simulink model "big2"  (R2023b)
settings: Solver=VariableStepAuto  StartTime=0.0  StopTime=500  RelTol=1e-3
libraries: simulink x2, aerolibasang x2, simulink_extras x2, aerolibanim x1
(part 1 of 3)
settings Model: Creator=TADTAWAN  LastModifiedBy=TADTAWAN

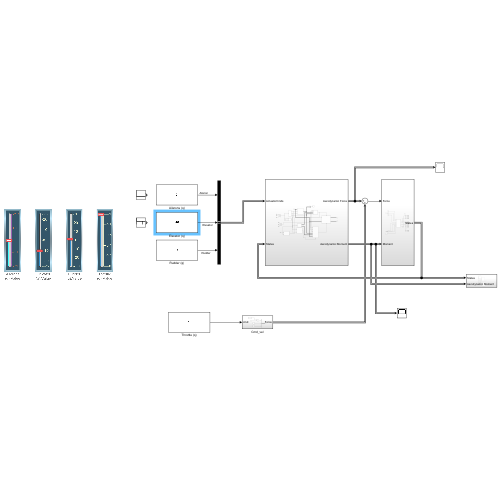
[thumbnail: Simulink's stored preview of the top-level diagram]
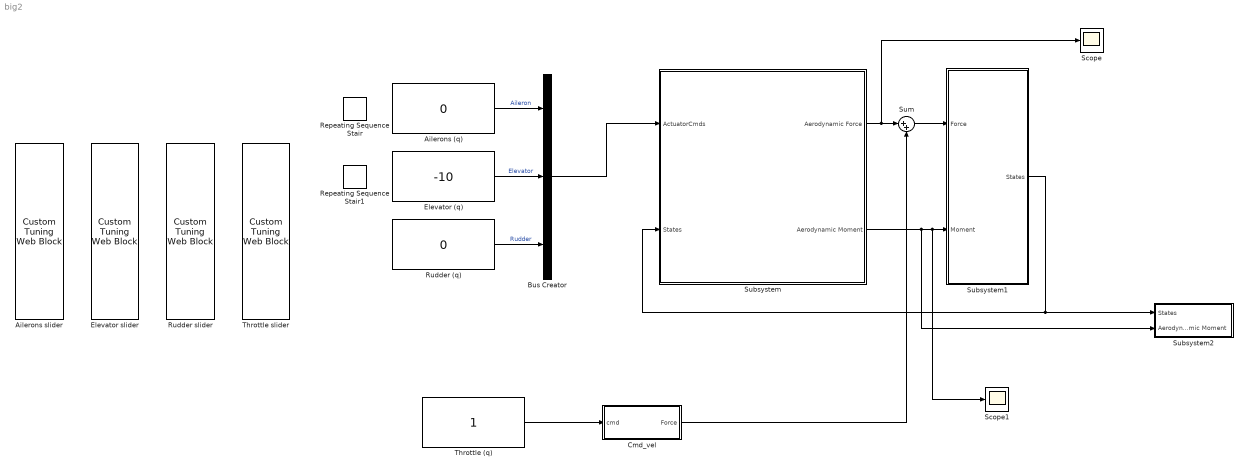
== system big2 ==
  Ailerons (q) : Constant  Value=0
  Ailerons slider : CustomTuningWebBlock  LabelPosition=Bottom  ShowInitialText=on  Configuration="{\"components\":[{\"name\":\"LinearScaleComponent\",\"settings\":{\"bounds\":{\"max\":21.5,\"min\":-21.5,\"tickInterval\":\"auto\"},\"internalTickHeightScaleFactor\":0.5,\"labelColor\":[181,82,43],\"labelFont\":{\"font\":\"Arial\",\"fontSize\":12},\"labelOffset\":0.05,\"labelTransparency\":1,\"needleImage\":{\"size\":[596,842],\"src\":\"data:image\\/svg+xml;base64,PD94bWwgdmVyc2lvbj0iMS4wIiBlbmNvZGluZz0idXRmLTgiPz4NCjwhLS0gR2VuZXJhdG9yOiBBZG9iZSBJbGx1c3RyYXRvciAyNS4wLjAsIFNWRyBFeHBvcnQgUGx1Zy1JbiAuIFNWRyBWZXJzaW9uOiA2LjAwIEJ1aWxkIDApICAtLT4NCjxzdmcgdmVyc2lvbj0iMS4xIg0KCSBpZD0ic3ZnOCIgeG1sbnM6Y2M9Imh0dHA6Ly9jcmVhdGl2ZWNvbW1vbnMub3JnL25zIyIgeG1sbnM6ZGM9Imh0dHA6Ly9wdXJsLm9yZy9kYy9lbGVtZW50cy8xLjEvIiB4bWxuczppbmtzY2FwZT0iaHR0cDovL3d3dy5pbmtzY2FwZS5vcmcvbmFtZXNw ...(+2420 chars)\",\"srcOrientation\":\"horizontal\"},\"needleOffset\":[0.0642123287671233,-0.8044596912521441],\"needleSize\":{\"height\":0.07668067226890757,\"width\":0.4337797619047619},\"position\":[0.03623949579831933,0.2829861111111111,0.6088789682539683,0.9196428571428571],\"referencePoint\":\"auto\",\"scaleColors\":[],\"scaleColorsSize\":0.2,\"scaleDirection\":\"BT\",\"showLabels\":1,\"showMinorTicks\":0,\"showSpanLine\":1,\"showTicks\":1,\"tickColor\":[150,61,168],\"tickTransparency\":1,\"valueBarColor\":[15,255,255],\"valueBarOffset\":-0.27,\"valueBarSize\":0.1,\"valueBarTransparency\":1}},{\"name\":\"BackgroundImageComponent\",\"settings\":{\"image\":{\"size\":[380,101],\"src\":\"data:image\\/svg+xml;base64,PHN2ZyB4bWxucz0iaHR0cDovL3d3dy53My5vcmcvMjAwMC9zdmciIHhtbG5zOnhsaW5rPSJodHRwOi8vd3d3LnczLm9yZy8xOTk5L3hsaW5rIiB2aWV3Qm94PSIwIDAgMzgwIDEwMSI+PGRlZnM+PHN0eWxlPi5jbHMtMXtmaWxsOiMwMDJiNDI7fS5jbHMtMntmaWxsOiM0MjcwODI7fS5jbHMtM3tmaWxsOnVybCgjcmFkaWFsLWdyYWRpZW50KTt9LmNscy00e2ZpbGw6I2M4YzhjODtzdHJva2U6IzAwMDt9PC9zdHlsZT48cmFkaWFsR3JhZGllbnQgaWQ9InJhZGlhbC1ncmFkaWVudCIgY3g9IjE5MCIgY3k9IjUwLjUiIHI9IjI2OS4yMSIgZ3JhZGllbnRVbml0cz0idXNlclNwYWNlT25Vc2UiPjxzdG9wIG9mZnNldD0iMC4wMSIgc3RvcC1jb2xvcj0iIzNlNGY1OCIvPjxzdG9wIG9mZnNldD0iMC4wNiIgc3RvcC1jb2xvcj0iIzQ0NTc2MSIvPjxzdG9wIG9mZnNldD0iMC4xNSIgc3RvcC1jb2xvcj0iIzU1NmE3NiIvPjxzdG9wIG9mZnNldD0iMC4yNSIgc3RvcC1jb2xvcj0iIzZkODg5NSIvPjxzdG9wIG9mZnNldD0iMC4zOCIgc3RvcC1jb2xvcj0iIzhmYjJjMyIvPjxzdG9wIG9mZnNldD0iMC41MiIgc3RvcC1jb2xvcj0iI2I2ZTRmYSIvPjxzdG9wIG9mZnNldD0iMSIgc3RvcC1jb2xvcj0iIzE1NDY1NyIvPjwvcmFkaWFsR3JhZGllbnQ+PC9kZWZzPjxnIGlkPSJmcmFtZSI+PGcgaWQ9IkxheWVyXzIiIGRhdGEtbmFtZT0iTGF5ZXIgMiI+PGcgaWQ9IkxheWVyXzEtMiIgZGF0YS1uYW1lPSJMYXllciAxLTIiPjxyZWN0IGlkPSJyZWN0MTAzNiIgY2xhc3M9ImNscy0xIiB4PSIxMSIgeT0iMTEiIHdpZHRoPSIzNTgiIGhlaWdodD0iNzkiLz48cGF0aCBpZD0icGF0aDEwMzgiIGNsYXNzPSJjbHMtMiIgZD0iTTgsOFY5M0gzNzJWOFpNMzY5LDkwSDExVjExSDM2OVoiLz48cGF0aCBpZD0icGF0aDEwNDAiIGNsYXNzPSJjbHMtMyIgZD0iTTAsMFYxMDFIMzgwVjBaTTM3Miw5M0g4VjhIMzcyWiIvPjwvZz48L2c+PC9nPjxnIGlkPSJ0cmFjayI+PHBhdGggaWQ9InJlY3QxNjExIiBjbGFzcz0iY2xzLTQiIGQ9Ik0zMy4zNywyNi41OUgzNDYuNjNjNCwwLDcuMjUsMi42LDcuMjUsNS44MWgwYzAsMy4yMS0zLjI1LDUuODItNy4yNSw1LjgySDMzLjM3Yy00LDAtNy4yNS0yLjYxLTcuMjUtNS44MmgwQzI2LjEyLDI5LjE5LDI5LjM3LDI2LjU5LDMzLjM3LDI2LjU5WiIvPjwvZz48L3N2Zz4=\",\"srcOrientation\":\"horizontal\"},\"position\":[0,0,1,1],\"scaleMode\":\"0\"}},{\"name\":\"ForegroundImageComponent\",\"settings\":{\"image\":{\"size\":[0,0],\"src\":\"default\",\"srcOrientation\":[]},\"isForeground\":1,\"position\":[0,0,1,1],\"scaleMode\":\"0\"}}],\"settings\":{\"BindingType\":\"param\",\"aspectRatio\":3.7777777777777777,\"backgroundColor\":[0,0,0,\"1\"],\"backgroundOffset\":0,\"backgroundOpacity\":1,\"fixedAspectRatio\":\"on\",\"foregroundColor\":[252,252,196],\"orientation\":\"vertical\",\"showBackgroundColor\":false,\"value\":0,\"version\":\"R2023a\"},\"type\":\"LinearGauge\"}"
  Bus Creator : BusCreator  Inputs=3
  Cmd_vel : Subsystem
  Elevator (q) : Constant  Value=-10
  Elevator slider : CustomTuningWebBlock  LabelPosition=Bottom  ShowInitialText=on  Configuration="{\"components\":[{\"name\":\"LinearScaleComponent\",\"settings\":{\"bounds\":{\"max\":25,\"min\":-25,\"tickInterval\":\"auto\"},\"internalTickHeightScaleFactor\":0.5,\"labelColor\":[255,255,200],\"labelFont\":{\"font\":\"Arial\",\"fontSize\":12},\"labelOffset\":0.05,\"labelTransparency\":1,\"needleImage\":{\"size\":[596,842],\"src\":\"data:image\\/svg+xml;base64,PD94bWwgdmVyc2lvbj0iMS4wIiBlbmNvZGluZz0idXRmLTgiPz4NCjwhLS0gR2VuZXJhdG9yOiBBZG9iZSBJbGx1c3RyYXRvciAyNS4wLjAsIFNWRyBFeHBvcnQgUGx1Zy1JbiAuIFNWRyBWZXJzaW9uOiA2LjAwIEJ1aWxkIDApICAtLT4NCjxzdmcgdmVyc2lvbj0iMS4xIg0KCSBpZD0ic3ZnOCIgeG1sbnM6Y2M9Imh0dHA6Ly9jcmVhdGl2ZWNvbW1vbnMub3JnL25zIyIgeG1sbnM6ZGM9Imh0dHA6Ly9wdXJsLm9yZy9kYy9lbGVtZW50cy8xLjEvIiB4bWxuczppbmtzY2FwZT0iaHR0cDovL3d3dy5pbmtzY2FwZS5vcmcvbmFtZXNw ...(+2420 chars)\",\"srcOrientation\":\"horizontal\"},\"needleOffset\":[0.0642123287671233,-0.8044596912521441],\"needleSize\":{\"height\":0.07668067226890757,\"width\":0.4337797619047619},\"position\":[0.03623949579831933,0.2829861111111111,0.6088789682539683,0.9196428571428571],\"referencePoint\":\"auto\",\"scaleColors\":[],\"scaleColorsSize\":0.2,\"scaleDirection\":\"BT\",\"showLabels\":1,\"showMinorTicks\":0,\"showSpanLine\":1,\"showTicks\":1,\"tickColor\":[252,252,197],\"tickTransparency\":1,\"valueBarColor\":[0,114,189],\"valueBarOffset\":-0.27,\"valueBarSize\":0.1,\"valueBarTransparency\":1}},{\"name\":\"BackgroundImageComponent\",\"settings\":{\"image\":{\"size\":[380,101],\"src\":\"data:image\\/svg+xml;base64,PHN2ZyB4bWxucz0iaHR0cDovL3d3dy53My5vcmcvMjAwMC9zdmciIHhtbG5zOnhsaW5rPSJodHRwOi8vd3d3LnczLm9yZy8xOTk5L3hsaW5rIiB2aWV3Qm94PSIwIDAgMzgwIDEwMSI+PGRlZnM+PHN0eWxlPi5jbHMtMXtmaWxsOiMwMDJiNDI7fS5jbHMtMntmaWxsOiM0MjcwODI7fS5jbHMtM3tmaWxsOnVybCgjcmFkaWFsLWdyYWRpZW50KTt9LmNscy00e2ZpbGw6I2M4YzhjODtzdHJva2U6IzAwMDt9PC9zdHlsZT48cmFkaWFsR3JhZGllbnQgaWQ9InJhZGlhbC1ncmFkaWVudCIgY3g9IjE5MCIgY3k9IjUwLjUiIHI9IjI2OS4yMSIgZ3JhZGllbnRVbml0cz0idXNlclNwYWNlT25Vc2UiPjxzdG9wIG9mZnNldD0iMC4wMSIgc3RvcC1jb2xvcj0iIzNlNGY1OCIvPjxzdG9wIG9mZnNldD0iMC4wNiIgc3RvcC1jb2xvcj0iIzQ0NTc2MSIvPjxzdG9wIG9mZnNldD0iMC4xNSIgc3RvcC1jb2xvcj0iIzU1NmE3NiIvPjxzdG9wIG9mZnNldD0iMC4yNSIgc3RvcC1jb2xvcj0iIzZkODg5NSIvPjxzdG9wIG9mZnNldD0iMC4zOCIgc3RvcC1jb2xvcj0iIzhmYjJjMyIvPjxzdG9wIG9mZnNldD0iMC41MiIgc3RvcC1jb2xvcj0iI2I2ZTRmYSIvPjxzdG9wIG9mZnNldD0iMSIgc3RvcC1jb2xvcj0iIzE1NDY1NyIvPjwvcmFkaWFsR3JhZGllbnQ+PC9kZWZzPjxnIGlkPSJmcmFtZSI+PGcgaWQ9IkxheWVyXzIiIGRhdGEtbmFtZT0iTGF5ZXIgMiI+PGcgaWQ9IkxheWVyXzEtMiIgZGF0YS1uYW1lPSJMYXllciAxLTIiPjxyZWN0IGlkPSJyZWN0MTAzNiIgY2xhc3M9ImNscy0xIiB4PSIxMSIgeT0iMTEiIHdpZHRoPSIzNTgiIGhlaWdodD0iNzkiLz48cGF0aCBpZD0icGF0aDEwMzgiIGNsYXNzPSJjbHMtMiIgZD0iTTgsOFY5M0gzNzJWOFpNMzY5LDkwSDExVjExSDM2OVoiLz48cGF0aCBpZD0icGF0aDEwNDAiIGNsYXNzPSJjbHMtMyIgZD0iTTAsMFYxMDFIMzgwVjBaTTM3Miw5M0g4VjhIMzcyWiIvPjwvZz48L2c+PC9nPjxnIGlkPSJ0cmFjayI+PHBhdGggaWQ9InJlY3QxNjExIiBjbGFzcz0iY2xzLTQiIGQ9Ik0zMy4zNywyNi41OUgzNDYuNjNjNCwwLDcuMjUsMi42LDcuMjUsNS44MWgwYzAsMy4yMS0zLjI1LDUuODItNy4yNSw1LjgySDMzLjM3Yy00LDAtNy4yNS0yLjYxLTcuMjUtNS44MmgwQzI2LjEyLDI5LjE5LDI5LjM3LDI2LjU5LDMzLjM3LDI2LjU5WiIvPjwvZz48L3N2Zz4=\",\"srcOrientation\":\"horizontal\"},\"position\":[0,0,1,1],\"scaleMode\":\"0\"}},{\"name\":\"ForegroundImageComponent\",\"settings\":{\"image\":{\"size\":[0,0],\"src\":\"default\",\"srcOrientation\":[]},\"isForeground\":1,\"position\":[0,0,1,1],\"scaleMode\":\"0\"}}],\"settings\":{\"BindingType\":\"param\",\"aspectRatio\":3.7777777777777777,\"backgroundColor\":[0,0,0,\"1\"],\"backgroundOffset\":0,\"backgroundOpacity\":1,\"fixedAspectRatio\":\"on\",\"foregroundColor\":[252,252,196],\"orientation\":\"vertical\",\"showBackgroundColor\":false,\"value\":0,\"version\":\"R2023a\"},\"type\":\"LinearGauge\"}"
  Repeating Sequence Stair : simulink/Sources/Repeating Sequence Stair  OutValues=[0 0 0 0 0 0 0 0 0 0 0 0 0 0 0 0 0 0 0 0 0 0 0 0 0 0 0 0 0 0 0 0 0].'  tsamp=8  OutMin=[]  OutMax=[]  OutDataTypeStr=double  OutputDataTypeScalingMode=double  OutDataType=fixdt(0,8)  ConRadixGroup=Best Precision: Vector-wise  OutScaling=2^-12
  Repeating Sequence Stair1 : simulink/Sources/Repeating Sequence Stair  OutValues=[25 0 0 0 0 0 0 0 0 0 0 0 0 0 0 0 0 0 0 0 0 0 0 0 0 0 0 0 0 -25 0 0 0 0 0 0 0 0 0 0 0 0 0 0 0].'  tsamp=5  OutMin=[]  OutMax=[]  OutDataTypeStr=double  OutputDataTypeScalingMode=double  OutDataType=fixdt(0,8)  ConRadixGroup=Best Precision: Vector-wise  OutScaling=2^-12
  Rudder (q) : Constant  Value=0
  Rudder slider : CustomTuningWebBlock  LabelPosition=Bottom  ShowInitialText=on  Configuration="{\"components\":[{\"name\":\"LinearScaleComponent\",\"settings\":{\"bounds\":{\"max\":30,\"min\":-30,\"tickInterval\":\"auto\"},\"internalTickHeightScaleFactor\":0.5,\"labelColor\":[255,255,200],\"labelFont\":{\"font\":\"Arial\",\"fontSize\":12},\"labelOffset\":0.05,\"labelTransparency\":1,\"needleImage\":{\"size\":[596,842],\"src\":\"data:image\\/svg+xml;base64,PD94bWwgdmVyc2lvbj0iMS4wIiBlbmNvZGluZz0idXRmLTgiPz4NCjwhLS0gR2VuZXJhdG9yOiBBZG9iZSBJbGx1c3RyYXRvciAyNS4wLjAsIFNWRyBFeHBvcnQgUGx1Zy1JbiAuIFNWRyBWZXJzaW9uOiA2LjAwIEJ1aWxkIDApICAtLT4NCjxzdmcgdmVyc2lvbj0iMS4xIg0KCSBpZD0ic3ZnOCIgeG1sbnM6Y2M9Imh0dHA6Ly9jcmVhdGl2ZWNvbW1vbnMub3JnL25zIyIgeG1sbnM6ZGM9Imh0dHA6Ly9wdXJsLm9yZy9kYy9lbGVtZW50cy8xLjEvIiB4bWxuczppbmtzY2FwZT0iaHR0cDovL3d3dy5pbmtzY2FwZS5vcmcvbmFtZXNw ...(+2420 chars)\",\"srcOrientation\":\"Right\"},\"needleOffset\":[-0.21513706793802145,-0.7877922077922078],\"needleSize\":{\"height\":0.07666301169590643,\"width\":0.43370508054522927},\"position\":[0.03623949579831933,0.2829861111111111,0.6088789682539683,0.9196428571428571],\"referencePoint\":\"auto\",\"scaleColors\":[],\"scaleColorsSize\":0.2,\"scaleDirection\":\"BT\",\"showLabels\":1,\"showMinorTicks\":0,\"showSpanLine\":1,\"showTicks\":1,\"tickColor\":[252,252,197],\"tickTransparency\":1,\"valueBarColor\":[0,114,189],\"valueBarOffset\":-0.27,\"valueBarSize\":0.1,\"valueBarTransparency\":1}},{\"name\":\"BackgroundImageComponent\",\"settings\":{\"image\":{\"size\":[380,101],\"src\":\"data:image\\/svg+xml;base64,PHN2ZyB4bWxucz0iaHR0cDovL3d3dy53My5vcmcvMjAwMC9zdmciIHhtbG5zOnhsaW5rPSJodHRwOi8vd3d3LnczLm9yZy8xOTk5L3hsaW5rIiB2aWV3Qm94PSIwIDAgMzgwIDEwMSI+PGRlZnM+PHN0eWxlPi5jbHMtMXtmaWxsOiMwMDJiNDI7fS5jbHMtMntmaWxsOiM0MjcwODI7fS5jbHMtM3tmaWxsOnVybCgjcmFkaWFsLWdyYWRpZW50KTt9LmNscy00e2ZpbGw6I2M4YzhjODtzdHJva2U6IzAwMDt9PC9zdHlsZT48cmFkaWFsR3JhZGllbnQgaWQ9InJhZGlhbC1ncmFkaWVudCIgY3g9IjE5MCIgY3k9IjUwLjUiIHI9IjI2OS4yMSIgZ3JhZGllbnRVbml0cz0idXNlclNwYWNlT25Vc2UiPjxzdG9wIG9mZnNldD0iMC4wMSIgc3RvcC1jb2xvcj0iIzNlNGY1OCIvPjxzdG9wIG9mZnNldD0iMC4wNiIgc3RvcC1jb2xvcj0iIzQ0NTc2MSIvPjxzdG9wIG9mZnNldD0iMC4xNSIgc3RvcC1jb2xvcj0iIzU1NmE3NiIvPjxzdG9wIG9mZnNldD0iMC4yNSIgc3RvcC1jb2xvcj0iIzZkODg5NSIvPjxzdG9wIG9mZnNldD0iMC4zOCIgc3RvcC1jb2xvcj0iIzhmYjJjMyIvPjxzdG9wIG9mZnNldD0iMC41MiIgc3RvcC1jb2xvcj0iI2I2ZTRmYSIvPjxzdG9wIG9mZnNldD0iMSIgc3RvcC1jb2xvcj0iIzE1NDY1NyIvPjwvcmFkaWFsR3JhZGllbnQ+PC9kZWZzPjxnIGlkPSJmcmFtZSI+PGcgaWQ9IkxheWVyXzIiIGRhdGEtbmFtZT0iTGF5ZXIgMiI+PGcgaWQ9IkxheWVyXzEtMiIgZGF0YS1uYW1lPSJMYXllciAxLTIiPjxyZWN0IGlkPSJyZWN0MTAzNiIgY2xhc3M9ImNscy0xIiB4PSIxMSIgeT0iMTEiIHdpZHRoPSIzNTgiIGhlaWdodD0iNzkiLz48cGF0aCBpZD0icGF0aDEwMzgiIGNsYXNzPSJjbHMtMiIgZD0iTTgsOFY5M0gzNzJWOFpNMzY5LDkwSDExVjExSDM2OVoiLz48cGF0aCBpZD0icGF0aDEwNDAiIGNsYXNzPSJjbHMtMyIgZD0iTTAsMFYxMDFIMzgwVjBaTTM3Miw5M0g4VjhIMzcyWiIvPjwvZz48L2c+PC9nPjxnIGlkPSJ0cmFjayI+PHBhdGggaWQ9InJlY3QxNjExIiBjbGFzcz0iY2xzLTQiIGQ9Ik0zMy4zNywyNi41OUgzNDYuNjNjNCwwLDcuMjUsMi42LDcuMjUsNS44MWgwYzAsMy4yMS0zLjI1LDUuODItNy4yNSw1LjgySDMzLjM3Yy00LDAtNy4yNS0yLjYxLTcuMjUtNS44MmgwQzI2LjEyLDI5LjE5LDI5LjM3LDI2LjU5LDMzLjM3LDI2LjU5WiIvPjwvZz48L3N2Zz4=\",\"srcOrientation\":\"horizontal\"},\"position\":[0,0,1,1],\"scaleMode\":\"0\"}},{\"name\":\"ForegroundImageComponent\",\"settings\":{\"image\":{\"size\":[0,0],\"src\":\"default\",\"srcOrientation\":[]},\"isForeground\":1,\"position\":[0,0,1,1],\"scaleMode\":\"0\"}}],\"settings\":{\"BindingType\":\"param\",\"aspectRatio\":3.7777777777777777,\"backgroundColor\":[0,0,0,\"1\"],\"backgroundOffset\":0,\"backgroundOpacity\":1,\"fixedAspectRatio\":\"on\",\"foregroundColor\":[252,252,196],\"orientation\":\"vertical\",\"showBackgroundColor\":false,\"value\":0,\"version\":\"R2023a\"},\"type\":\"LinearGauge\"}"
  Scope : Scope
  Scope1 : Scope
  Subsystem : Subsystem
  Subsystem1 : Subsystem
  Subsystem2 : Subsystem
  Sum : Sum  Inputs=|++
  Throttle (q) : Constant
  Throttle slider : CustomTuningWebBlock  LabelPosition=Bottom  ShowInitialText=on  Configuration="{\"components\":[{\"name\":\"LinearScaleComponent\",\"settings\":{\"bounds\":{\"max\":1,\"min\":0,\"tickInterval\":\"auto\"},\"internalTickHeightScaleFactor\":0.5,\"labelColor\":[255,255,200],\"labelFont\":{\"font\":\"Arial\",\"fontSize\":12},\"labelOffset\":0.05,\"labelTransparency\":1,\"needleImage\":{\"size\":[596,842],\"src\":\"data:image\\/svg+xml;base64,PD94bWwgdmVyc2lvbj0iMS4wIiBlbmNvZGluZz0idXRmLTgiPz4NCjwhLS0gR2VuZXJhdG9yOiBBZG9iZSBJbGx1c3RyYXRvciAyNS4wLjAsIFNWRyBFeHBvcnQgUGx1Zy1JbiAuIFNWRyBWZXJzaW9uOiA2LjAwIEJ1aWxkIDApICAtLT4NCjxzdmcgdmVyc2lvbj0iMS4xIg0KCSBpZD0ic3ZnOCIgeG1sbnM6Y2M9Imh0dHA6Ly9jcmVhdGl2ZWNvbW1vbnMub3JnL25zIyIgeG1sbnM6ZGM9Imh0dHA6Ly9wdXJsLm9yZy9kYy9lbGVtZW50cy8xLjEvIiB4bWxuczppbmtzY2FwZT0iaHR0cDovL3d3dy5pbmtzY2FwZS5vcmcvbmFtZXNw ...(+2420 chars)\",\"srcOrientation\":\"horizontal\"},\"needleOffset\":[0.0642123287671233,-0.8044596912521441],\"needleSize\":{\"height\":0.07668067226890757,\"width\":0.4337797619047619},\"position\":[0.03623949579831933,0.2829861111111111,0.6088789682539683,0.9196428571428571],\"referencePoint\":\"auto\",\"scaleColors\":[],\"scaleColorsSize\":0.2,\"scaleDirection\":\"BT\",\"showLabels\":1,\"showMinorTicks\":0,\"showSpanLine\":1,\"showTicks\":1,\"tickColor\":[252,252,197],\"tickTransparency\":1,\"valueBarColor\":[0,114,189],\"valueBarOffset\":-0.27,\"valueBarSize\":0.1,\"valueBarTransparency\":1}},{\"name\":\"BackgroundImageComponent\",\"settings\":{\"image\":{\"size\":[380,101],\"src\":\"data:image\\/svg+xml;base64,PHN2ZyB4bWxucz0iaHR0cDovL3d3dy53My5vcmcvMjAwMC9zdmciIHhtbG5zOnhsaW5rPSJodHRwOi8vd3d3LnczLm9yZy8xOTk5L3hsaW5rIiB2aWV3Qm94PSIwIDAgMzgwIDEwMSI+PGRlZnM+PHN0eWxlPi5jbHMtMXtmaWxsOiMwMDJiNDI7fS5jbHMtMntmaWxsOiM0MjcwODI7fS5jbHMtM3tmaWxsOnVybCgjcmFkaWFsLWdyYWRpZW50KTt9LmNscy00e2ZpbGw6I2M4YzhjODtzdHJva2U6IzAwMDt9PC9zdHlsZT48cmFkaWFsR3JhZGllbnQgaWQ9InJhZGlhbC1ncmFkaWVudCIgY3g9IjE5MCIgY3k9IjUwLjUiIHI9IjI2OS4yMSIgZ3JhZGllbnRVbml0cz0idXNlclNwYWNlT25Vc2UiPjxzdG9wIG9mZnNldD0iMC4wMSIgc3RvcC1jb2xvcj0iIzNlNGY1OCIvPjxzdG9wIG9mZnNldD0iMC4wNiIgc3RvcC1jb2xvcj0iIzQ0NTc2MSIvPjxzdG9wIG9mZnNldD0iMC4xNSIgc3RvcC1jb2xvcj0iIzU1NmE3NiIvPjxzdG9wIG9mZnNldD0iMC4yNSIgc3RvcC1jb2xvcj0iIzZkODg5NSIvPjxzdG9wIG9mZnNldD0iMC4zOCIgc3RvcC1jb2xvcj0iIzhmYjJjMyIvPjxzdG9wIG9mZnNldD0iMC41MiIgc3RvcC1jb2xvcj0iI2I2ZTRmYSIvPjxzdG9wIG9mZnNldD0iMSIgc3RvcC1jb2xvcj0iIzE1NDY1NyIvPjwvcmFkaWFsR3JhZGllbnQ+PC9kZWZzPjxnIGlkPSJmcmFtZSI+PGcgaWQ9IkxheWVyXzIiIGRhdGEtbmFtZT0iTGF5ZXIgMiI+PGcgaWQ9IkxheWVyXzEtMiIgZGF0YS1uYW1lPSJMYXllciAxLTIiPjxyZWN0IGlkPSJyZWN0MTAzNiIgY2xhc3M9ImNscy0xIiB4PSIxMSIgeT0iMTEiIHdpZHRoPSIzNTgiIGhlaWdodD0iNzkiLz48cGF0aCBpZD0icGF0aDEwMzgiIGNsYXNzPSJjbHMtMiIgZD0iTTgsOFY5M0gzNzJWOFpNMzY5LDkwSDExVjExSDM2OVoiLz48cGF0aCBpZD0icGF0aDEwNDAiIGNsYXNzPSJjbHMtMyIgZD0iTTAsMFYxMDFIMzgwVjBaTTM3Miw5M0g4VjhIMzcyWiIvPjwvZz48L2c+PC9nPjxnIGlkPSJ0cmFjayI+PHBhdGggaWQ9InJlY3QxNjExIiBjbGFzcz0iY2xzLTQiIGQ9Ik0zMy4zNywyNi41OUgzNDYuNjNjNCwwLDcuMjUsMi42LDcuMjUsNS44MWgwYzAsMy4yMS0zLjI1LDUuODItNy4yNSw1LjgySDMzLjM3Yy00LDAtNy4yNS0yLjYxLTcuMjUtNS44MmgwQzI2LjEyLDI5LjE5LDI5LjM3LDI2LjU5LDMzLjM3LDI2LjU5WiIvPjwvZz48L3N2Zz4=\",\"srcOrientation\":\"horizontal\"},\"position\":[0,0,1,1],\"scaleMode\":\"0\"}},{\"name\":\"ForegroundImageComponent\",\"settings\":{\"image\":{\"size\":[0,0],\"src\":\"default\",\"srcOrientation\":[]},\"isForeground\":1,\"position\":[0,0,1,1],\"scaleMode\":\"0\"}}],\"settings\":{\"BindingType\":\"param\",\"aspectRatio\":3.7777777777777777,\"backgroundColor\":[0,0,0,\"1\"],\"backgroundOffset\":0,\"backgroundOpacity\":1,\"fixedAspectRatio\":\"on\",\"foregroundColor\":[252,252,196],\"orientation\":\"vertical\",\"showBackgroundColor\":false,\"value\":0,\"version\":\"R2023a\"},\"type\":\"LinearGauge\"}"
  wires:
  Throttle (q)/1 -> Cmd_vel/1(cmd)
  Bus Creator/1 -> Subsystem/1(ActuatorCmds)
  Subsystem1/1(States) -> Subsystem/2(States), Subsystem2/1(States)
  Cmd_vel/1(Force) -> Sum/2
  Sum/1 -> Subsystem1/1(Force)
  Rudder (q)/1 -> Bus Creator/3  "Rudder"
  Subsystem/1(Aerodynamic Force) -> Scope/1, Sum/1
  Subsystem/2(Aerodynamic Moment) -> Subsystem2/2(Aerodynamic Moment), Scope1/1, Subsystem1/2(Moment)
  Elevator (q)/1 -> Bus Creator/2  "Elevator"
  Ailerons (q)/1 -> Bus Creator/1  "Aileron"

== system big2/Cmd_vel ==
  cmd : Inport
  Bus Creator : BusCreator  Inputs=3
  Constant : Constant  Value=0
  Constant1 : Constant  Value=0
  Engine Power : Constant  Value=20500
  F_x : Product
  Force : Outport
  wires:
  Engine Power/1 -> F_x/1
  cmd/1 -> F_x/2
  F_x/1 -> Bus Creator/1  "F_x"
  Constant/1 -> Bus Creator/2  "F_y"
  Constant1/1 -> Bus Creator/3  "F_z"
  Bus Creator/1 -> Force/1

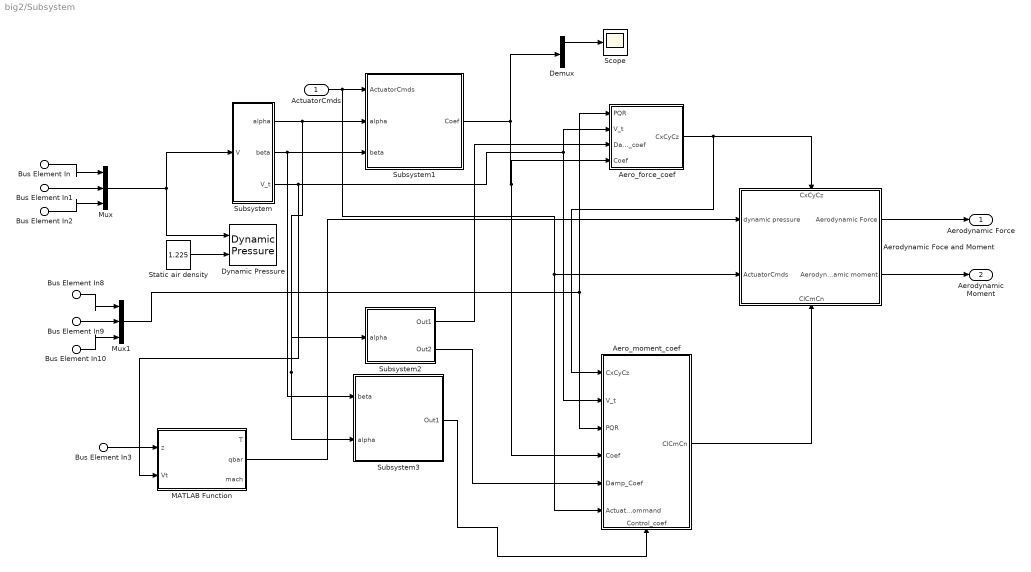
== system big2/Subsystem ==
  ActuatorCmds : Inport
  Bus Element In : Inport  Port=2  PortName=States  Element=U
  Bus Element In1 : Inport  Port=2  PortName=States  Element=V
  Bus Element In2 : Inport  Port=2  PortName=States  Element=W
  Bus Element In8 : Inport  Port=2  PortName=States  Element=p
  Bus Element In9 : Inport  Port=2  PortName=States  Element=q
  Bus Element In10 : Inport  Port=2  PortName=States  Element=r
  Bus Element In3 : Inport  Port=2  PortName=States  Element=Ze
  Aero_force_coef : Subsystem
  Aero_moment_coef : Subsystem
      settings: PortSchema="{\"entries\":[{\"content\":{\"sides\":[{\"content\":{\"connectorIds\":[\"In1\",\"In2\",\"In3\",\"In4\",\"In5\",\"In6\"]},\"type\":\"ConnectorPlacement.EquallySpacedRectSide\",\"uuid\":\"17debfaa-879f-41a8-9d58-1f255e45b172\"},{\"content\":{\"connectorIds\":[\"Out1\"],\"side\":\"RIGHT\"},\"type\":\"ConnectorPlacement.EquallySpacedRectSide\",\"uuid\":\"f07a405c-0f85-43ee-be51-ba40d2608d18\"},{\"content\":{\"side\":\"TOP\"},\"type\":\"ConnectorPlacement.EquallySpacedRectSide\",\"uuid\":\"8673e22a-5761-41aa-9cd5-8d56fc2beb8a\"},{\"content\":{\"connectorIds\":[\"In7\"],\"side\":\"BOTTOM\"},\"type\":\"ConnectorPlacement.EquallySpacedRectSide\",\"uuid\":\"a74aac7f-3bc3-4068-9fca-4bb700d9041f\"}]},\"type\":\"ConnectorPlacement.EquallySpacedConnector\",\"uuid\":\"42287ef6-e7dd-4b60-8942-44cb4f2566c7\"}],\"packageUris\":[\"http://schema.mathworks.com/mf0/Connector/R2020b\"],\"version\":\"1.0\"}"
  Aerodynamic Foce and Moment : Subsystem
      settings: PortSchema="{\"entries\":[{\"content\":{\"sides\":[{\"content\":{\"connectorIds\":[\"In1\",\"In2\"]},\"type\":\"ConnectorPlacement.EquallySpacedRectSide\",\"uuid\":\"ab71a591-92c3-4a8b-addc-090922ce6fb0\"},{\"content\":{\"connectorIds\":[\"Out1\",\"Out2\"],\"side\":\"RIGHT\"},\"type\":\"ConnectorPlacement.EquallySpacedRectSide\",\"uuid\":\"1820ed69-80c2-44ce-a026-73df58491777\"},{\"content\":{\"connectorIds\":[\"In3\"],\"side\":\"TOP\"},\"type\":\"ConnectorPlacement.EquallySpacedRectSide\",\"uuid\":\"870b67ff-c9d8-4b48-8001-55133f95ea6a\"},{\"content\":{\"connectorIds\":[\"In4\"],\"side\":\"BOTTOM\"},\"type\":\"ConnectorPlacement.EquallySpacedRectSide\",\"uuid\":\"51f11529-3a1c-4e22-ab27-30b6bff5f544\"}]},\"type\":\"ConnectorPlacement.EquallySpacedConnector\",\"uuid\":\"5a950543-611d-42e3-87a9-2998e260972e\"}],\"packageUris\":[\"http://schema.mathworks.com/mf0/Connector/R2020b\"],\"version\":\"1.0\"}"
  Demux : Demux  Outputs=6
  Dynamic Pressure : aerolibasang/Dynamic Pressure
  MATLAB Function : MATLAB Function  TreatAsAtomicUnit=on
  Mux : Mux  Inputs=3
  Mux1 : Mux  Inputs=3
  Scope : Scope
  Static air density : Constant  Value=1.225
  Subsystem : Subsystem
  Subsystem1 : Subsystem
  Subsystem2 : Subsystem
  Subsystem3 : Subsystem
  Aerodynamic Force : Outport
  Aerodynamic Moment : Outport  Port=2
  wires:
  Bus Element In1/1 -> Mux/2
  Bus Element In/1 -> Mux/1
  Bus Element In2/1 -> Mux/3
  Mux/1 -> Dynamic Pressure/1, Subsystem/1(V)
  ActuatorCmds/1 -> Aerodynamic Foce and Moment/2(ActuatorCmds), Aero_moment_coef/6(Actuatorcommand), Subsystem1/1(ActuatorCmds)
  Static air density/1 -> Dynamic Pressure/2
  Subsystem1/1(Coef) -> Aero_moment_coef/4(Coef), Aero_force_coef/4(Coef), Demux/1
  Aerodynamic Foce and Moment/1(Aerodynamic Force) -> Aerodynamic Force/1
  Aerodynamic Foce and Moment/2(Aerodynamic moment) -> Aerodynamic Moment/1
  Demux/1 -> Scope/1
  Subsystem/3(V_t) -> MATLAB Function/2(Vt), Aero_moment_coef/2(V_t), Aero_force_coef/2(V_t)
  Mux1/1 -> Aero_moment_coef/3(PQR), Aero_force_coef/1(PQR)
  Bus Element In8/1 -> Mux1/1
  Bus Element In9/1 -> Mux1/2
  Bus Element In10/1 -> Mux1/3
  Aero_force_coef/1(CxCyCz) -> Aero_moment_coef/1(CxCyCz), Aerodynamic Foce and Moment/3(CxCyCz)
  Subsystem2/1(Out1) -> Aero_force_coef/3(Damp_coef)
  Subsystem2/2(Out2) -> Aero_moment_coef/5(Damp_Coef)
  Aero_moment_coef/1(ClCmCn) -> Aerodynamic Foce and Moment/4(ClCmCn)
  Subsystem/1(alpha) -> Subsystem3/2(alpha), Subsystem2/1(alpha), Subsystem1/2(alpha)
  Subsystem/2(beta) -> Subsystem3/1(beta), Subsystem1/3(beta)
  Subsystem3/1(Out1) -> Aero_moment_coef/7(Control_coef)
  Bus Element In3/1 -> MATLAB Function/1(z)
  MATLAB Function/2(qbar) -> Aerodynamic Foce and Moment/1(dynamic pressure)

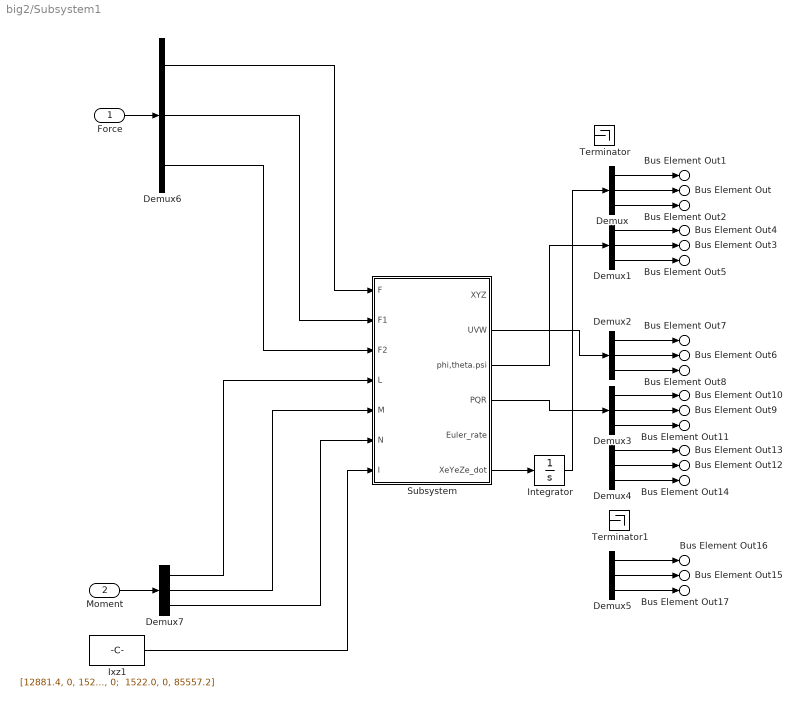
== system big2/Subsystem1 ==
  Force : Inport
  Moment : Inport  Port=2
  Demux{,1..7} (8 alike) : Demux  Outputs=3
  Integrator : Integrator  InitialCondition=[0;0;-1500]
  Ixz1 : Constant  Value=|
      | [12881.4, 0, 1522.0;
      |  0, 75696.9, 0;
      |  1522.0, 0, 85557.2]
  Subsystem : Subsystem
  Terminator : Terminator
  Terminator1 : Terminator
  Bus Element Out : Outport  PortName=States  Element=Ye
  Bus Element Out1 : Outport  PortName=States  Element=Xe
  Bus Element Out2 : Outport  PortName=States  Element=Ze
  Bus Element Out3 : Outport  PortName=States  Element=theta
  Bus Element Out4 : Outport  PortName=States  Element=phi
  Bus Element Out5 : Outport  PortName=States  Element=psi
  Bus Element Out6 : Outport  PortName=States  Element=V
  Bus Element Out7 : Outport  PortName=States  Element=U
  Bus Element Out8 : Outport  PortName=States  Element=W
  Bus Element Out9 : Outport  PortName=States  Element=q
  Bus Element Out10 : Outport  PortName=States  Element=p
  Bus Element Out11 : Outport  PortName=States  Element=r
  Bus Element Out12 : Outport  PortName=States  Element=q_dot
  Bus Element Out13 : Outport  PortName=States  Element=p_dot
  Bus Element Out14 : Outport  PortName=States  Element=r_dot
  Bus Element Out15 : Outport  PortName=States  Element=Aye
  Bus Element Out16 : Outport  PortName=States  Element=Axe
  Bus Element Out17 : Outport  PortName=States  Element=Aze
  wires:
  Demux/2 -> Bus Element Out/1
  Demux/1 -> Bus Element Out1/1
  Demux/3 -> Bus Element Out2/1
  Demux1/3 -> Bus Element Out5/1
  Demux1/2 -> Bus Element Out3/1
  Demux1/1 -> Bus Element Out4/1
  Demux2/1 -> Bus Element Out7/1
  Demux2/3 -> Bus Element Out8/1
  Demux2/2 -> Bus Element Out6/1
  Demux3/1 -> Bus Element Out10/1
  Demux3/3 -> Bus Element Out11/1
  Demux3/2 -> Bus Element Out9/1
  Demux4/1 -> Bus Element Out13/1
  Demux4/3 -> Bus Element Out14/1
  Demux4/2 -> Bus Element Out12/1
  Demux5/1 -> Bus Element Out16/1
  Demux5/3 -> Bus Element Out17/1
  Demux5/2 -> Bus Element Out15/1
  Force/1 -> Demux6/1
  Moment/1 -> Demux7/1
  Demux6/1 -> Subsystem/1(F)
  Demux6/2 -> Subsystem/2(F1)
  Demux6/3 -> Subsystem/3(F2)
  Demux7/1 -> Subsystem/4(L)
  Demux7/2 -> Subsystem/5(M)
  Demux7/3 -> Subsystem/6(N)
  Ixz1/1 -> Subsystem/7(I)
  Subsystem/4(PQR) -> Demux3/1
  Subsystem/3(phi,theta.psi) -> Demux1/1
  Subsystem/2(UVW) -> Demux2/1
  Subsystem/6(XeYeZe_dot) -> Integrator/1
  Integrator/1 -> Demux/1

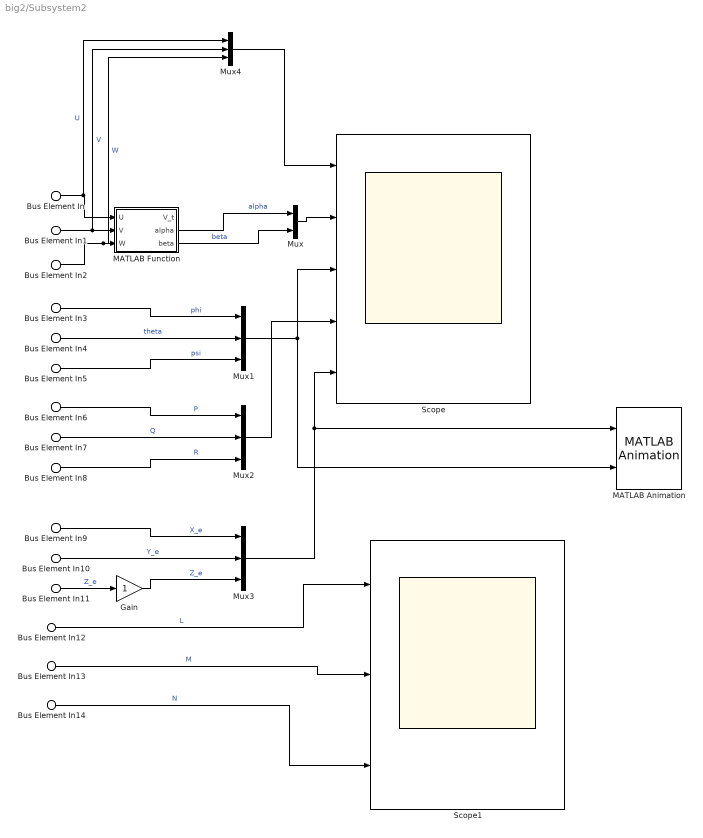
== system big2/Subsystem2 ==
  Bus Element In : Inport  PortName=States  Element=U
  Bus Element In2 : Inport  PortName=States  Element=W
  Bus Element In1 : Inport  PortName=States  Element=V
  Bus Element In3 : Inport  PortName=States  Element=phi
  Bus Element In4 : Inport  PortName=States  Element=theta
  Bus Element In5 : Inport  PortName=States  Element=psi
  Bus Element In6 : Inport  PortName=States  Element=p
  Bus Element In7 : Inport  PortName=States  Element=q
  Bus Element In8 : Inport  PortName=States  Element=r
  Bus Element In9 : Inport  PortName=States  Element=Xe
  Bus Element In10 : Inport  PortName=States  Element=Ye
  Bus Element In11 : Inport  PortName=States  Element=Ze
  Bus Element In12 : Inport  Port=2  PortName=Aerodynamic Moment  Element=L
  Bus Element In13 : Inport  Port=2  PortName=Aerodynamic Moment  Element=M
  Bus Element In14 : Inport  Port=2  PortName=Aerodynamic Moment  Element=N
  Gain : Gain
  MATLAB Animation : aerolibanim/MATLAB Animation  Tag=Matlab Animation 6 DOF  Vehicles=1  Geometries='astredwedge.mat'  BoundingBoxCoordinates=[-50,50,-50,50,-50,50]  CameraOffset=[-150,-50,0]  CameraViewAngle=3  SampleTime=0.2  FigurePosition=[-1919,64,1536,766]
  MATLAB Function : MATLAB Function  TreatAsAtomicUnit=on
  Mux : Mux  Inputs=2
  Mux{1..4} (4 alike) : Mux  Inputs=3
  Scope : Scope  NumInputPorts=5
  Scope1 : Scope  NumInputPorts=3
  wires:
  Bus Element In/1 -> Mux4/1, MATLAB Function/1(U)  "U"
  Bus Element In1/1 -> MATLAB Function/2(V), Mux4/2  "V"
  Bus Element In2/1 -> Mux4/3, MATLAB Function/3(W)  "W"
  MATLAB Function/2(alpha) -> Mux/1  "alpha"
  MATLAB Function/3(beta) -> Mux/2  "beta"
  Mux/1 -> Scope/2
  Bus Element In4/1 -> Mux1/2  "theta"
  Bus Element In3/1 -> Mux1/1  "phi"
  Bus Element In5/1 -> Mux1/3  "psi"
  Mux1/1 -> MATLAB Animation/2, Scope/3
  Bus Element In8/1 -> Mux2/3  "R"
  Bus Element In7/1 -> Mux2/2  "Q"
  Mux2/1 -> Scope/4
  Bus Element In6/1 -> Mux2/1  "P"
  Bus Element In11/1 -> Gain/1  "Z_e"
  Bus Element In10/1 -> Mux3/2  "Y_e"
  Bus Element In9/1 -> Mux3/1  "X_e"
  Mux3/1 -> Scope/5, MATLAB Animation/1
  Bus Element In13/1 -> Scope1/2  "M"
  Bus Element In12/1 -> Scope1/1  "L"
  Bus Element In14/1 -> Scope1/3  "N"
  Gain/1 -> Mux3/3  "Z_e"
  Mux4/1 -> Scope/1

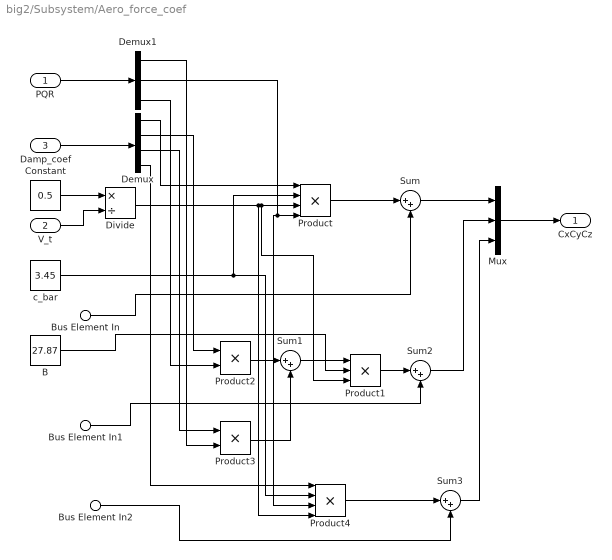
== system big2/Subsystem/Aero_force_coef ==
  PQR : Inport
  V_t : Inport  Port=2
  Damp_coef : Inport  Port=3
  Bus Element In : Inport  Port=4  PortName=Coef  Element=c_x
  Bus Element In1 : Inport  Port=4  PortName=Coef  Element=c_y
  Bus Element In2 : Inport  Port=4  PortName=Coef  Element=c_z
  B : Constant  Value=27.87
  Constant : Constant  Value=0.5
  Demux : Demux
  Demux1 : Demux  Outputs=3
  Divide : Product  Inputs=*/
  Mux : Mux  Inputs=3
  Product : Product  Inputs=4
  Product1 : Product  Inputs=3
  Product2 : Product
  Product3 : Product
  Product4 : Product  Inputs=4
  Sum{,1..3} (4 alike) : Sum  Inputs=|++
  c_bar : Constant  Value=3.45
  CxCyCz : Outport
  wires:
  V_t/1 -> Divide/2
  Constant/1 -> Divide/1
  Damp_coef/1 -> Demux/1
  PQR/1 -> Demux1/1
  Divide/1 -> Product1/3, Product/3, Product4/4
  Bus Element In/1 -> Sum/2
  c_bar/1 -> Product4/2, Product/2
  Demux1/2 -> Product/4, Product4/3
  Product/1 -> Sum/1
  Mux/1 -> CxCyCz/1
  Demux/2 -> Product2/1
  Demux/3 -> Product3/1
  Product2/1 -> Sum1/1
  Product3/1 -> Sum1/2
  Demux/1 -> Product/1
  Sum1/1 -> Product1/1
  B/1 -> Product1/2
  Product1/1 -> Sum2/1
  Bus Element In1/1 -> Sum2/2
  Sum2/1 -> Mux/2
  Sum/1 -> Mux/1
  Demux/4 -> Product4/1
  Product4/1 -> Sum3/1
  Bus Element In2/1 -> Sum3/2
  Sum3/1 -> Mux/3
  Demux1/3 -> Product2/2
  Demux1/1 -> Product3/2

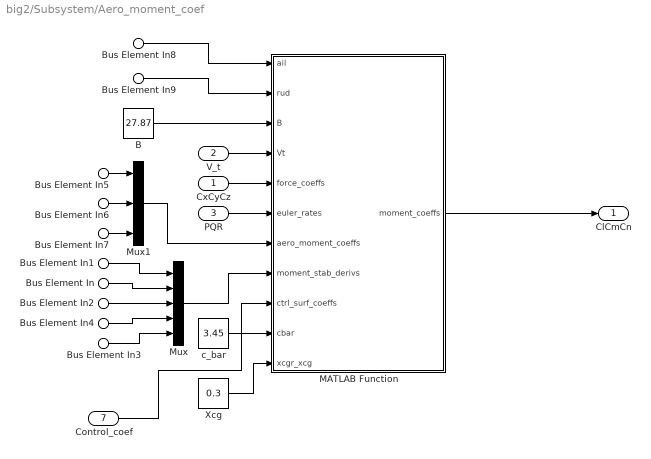
== system big2/Subsystem/Aero_moment_coef ==
  CxCyCz : Inport
  V_t : Inport  Port=2
  PQR : Inport  Port=3
  Bus Element In5 : Inport  Port=4  PortName=Coef  Element=c_l
  Bus Element In6 : Inport  Port=4  PortName=Coef  Element=c_m
  Bus Element In7 : Inport  Port=4  PortName=Coef  Element=c_n
  Bus Element In : Inport  Port=5  PortName=Damp_Coef  Element=Clp
  Bus Element In1 : Inport  Port=5  PortName=Damp_Coef  Element=Clr
  Bus Element In2 : Inport  Port=5  PortName=Damp_Coef  Element=Cmp
  Bus Element In3 : Inport  Port=5  PortName=Damp_Coef  Element=Cnp
  Bus Element In4 : Inport  Port=5  PortName=Damp_Coef  Element=Cnr
  Bus Element In8 : Inport  Port=6  PortName=Actuatorcommand  Element=Aileron
  Bus Element In9 : Inport  Port=6  PortName=Actuatorcommand  Element=Rudder
  Control_coef : Inport  Port=7
  B : Constant  Value=27.87
  MATLAB Function : MATLAB Function  TreatAsAtomicUnit=on
  Mux : Mux  Inputs=5
  Mux1 : Mux  Inputs=3
  Xcg : Constant  Value=0.3
  c_bar : Constant  Value=3.45
  ClCmCn : Outport
  wires:
  MATLAB Function/1(moment_coeffs) -> ClCmCn/1
  Mux/1 -> MATLAB Function/8(moment_stab_derivs)
  Bus Element In2/1 -> Mux/3
  Bus Element In/1 -> Mux/2
  Bus Element In1/1 -> Mux/1
  Bus Element In4/1 -> Mux/4
  Bus Element In3/1 -> Mux/5
  PQR/1 -> MATLAB Function/6(euler_rates)
  Bus Element In7/1 -> Mux1/3
  Bus Element In6/1 -> Mux1/2
  Bus Element In5/1 -> Mux1/1
  Mux1/1 -> MATLAB Function/7(aero_moment_coeffs)
  B/1 -> MATLAB Function/3(B)
  V_t/1 -> MATLAB Function/4(Vt)
  c_bar/1 -> MATLAB Function/10(cbar)
  Xcg/1 -> MATLAB Function/11(xcgr_xcg)
  Bus Element In8/1 -> MATLAB Function/1(ail)
  Bus Element In9/1 -> MATLAB Function/2(rud)
  CxCyCz/1 -> MATLAB Function/5(force_coeffs)
  Control_coef/1 -> MATLAB Function/9(ctrl_surf_coeffs)

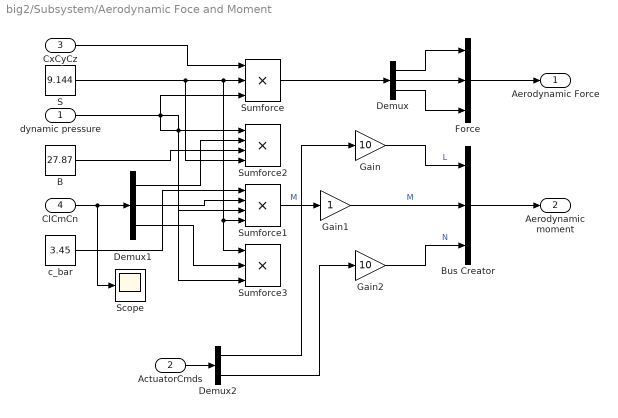
== system big2/Subsystem/Aerodynamic Foce and Moment ==
  dynamic pressure : Inport
  ActuatorCmds : Inport  Port=2
  CxCyCz : Inport  Port=3
  ClCmCn : Inport  Port=4
  B : Constant  Value=27.87
  Bus Creator : BusCreator  Inputs=3
  Demux : Demux  Outputs=3
  Demux1 : Demux  Outputs=3
  Demux2 : Demux  Outputs=3
  Force : BusCreator  Inputs=3
  Gain : Gain  Gain=10
  Gain1 : Gain
  Gain2 : Gain  Gain=10
  S : Constant  Value=9.144
  Scope : Scope
  Sumforce : Product  Inputs=3
  Sumforce1 : Product  Inputs=4
  Sumforce2 : Product  Inputs=4
  Sumforce3 : Product  Inputs=3
  c_bar : Constant  Value=3.45
  Aerodynamic Force : Outport
  Aerodynamic moment : Outport  Port=2
  wires:
  dynamic pressure/1 -> Sumforce/3, Sumforce3/3, Sumforce1/3, Sumforce2/1
  Force/1 -> Aerodynamic Force/1
  CxCyCz/1 -> Sumforce/1
  S/1 -> Sumforce2/4, Sumforce3/1, Sumforce1/4, Sumforce/2
  Sumforce/1 -> Demux/1
  Demux/1 -> Force/1
  Demux/2 -> Force/2
  Demux/3 -> Force/3
  ClCmCn/1 -> Scope/1, Demux1/1
  Demux1/2 -> Sumforce1/2
  Demux1/3 -> Sumforce3/2
  Demux1/1 -> Sumforce2/2
  B/1 -> Sumforce2/3
  c_bar/1 -> Sumforce1/1
  Sumforce1/1 -> Gain1/1  "M"
  Bus Creator/1 -> Aerodynamic moment/1
  Gain/1 -> Bus Creator/1  "L"
  Gain1/1 -> Bus Creator/2  "M"
  Gain2/1 -> Bus Creator/3  "N"
  ActuatorCmds/1 -> Demux2/1
  Demux2/1 -> Gain/1
  Demux2/3 -> Gain2/1

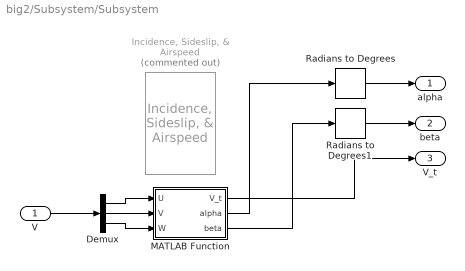
== system big2/Subsystem/Subsystem ==
  V : Inport
  Demux : Demux  Outputs=3
  "Incidence, Sideslip, & Airspeed" : aerolibasang/Incidence, Sideslip, & Airspeed  Commented=on
  MATLAB Function : MATLAB Function  TreatAsAtomicUnit=on
  Radians to Degrees : simulink_extras/Transformations/Radians to Degrees
  Radians to Degrees1 : simulink_extras/Transformations/Radians to Degrees
  alpha : Outport
  beta : Outport  Port=2
  V_t : Outport  Port=3
  wires:
  V/1 -> Demux/1
  Demux/1 -> MATLAB Function/1(U)
  Demux/2 -> MATLAB Function/2(V)
  Demux/3 -> MATLAB Function/3(W)
  Radians to Degrees/1 -> alpha/1
  Radians to Degrees1/1 -> beta/1
  MATLAB Function/3(beta) -> Radians to Degrees1/1
  MATLAB Function/2(alpha) -> Radians to Degrees/1
  MATLAB Function/1(V_t) -> V_t/1

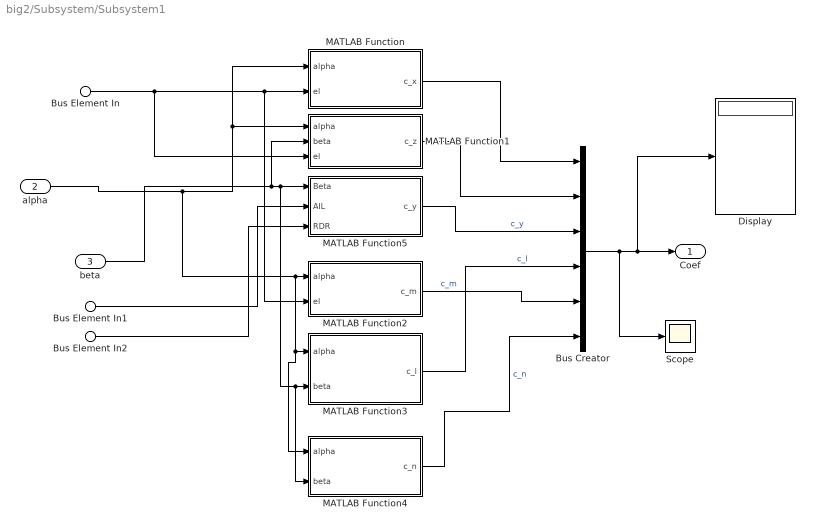
== system big2/Subsystem/Subsystem1 ==
  Bus Element In : Inport  PortName=ActuatorCmds  Element=Elevator
  Bus Element In1 : Inport  PortName=ActuatorCmds  Element=Aileron
  Bus Element In2 : Inport  PortName=ActuatorCmds  Element=Rudder
  alpha : Inport  Port=2
  beta : Inport  Port=3
  Bus Creator : BusCreator  Inputs=6
  Display : Display
  MATLAB Function : MATLAB Function  TreatAsAtomicUnit=on
  MATLAB Function1 : MATLAB Function  TreatAsAtomicUnit=on
  MATLAB Function2 : MATLAB Function  TreatAsAtomicUnit=on
  MATLAB Function3 : MATLAB Function  TreatAsAtomicUnit=on
  MATLAB Function4 : MATLAB Function  TreatAsAtomicUnit=on
  MATLAB Function5 : MATLAB Function  TreatAsAtomicUnit=on
  Scope : Scope
  Coef : Outport
  wires:
  Bus Element In1/1 -> MATLAB Function5/2(AIL)
  Bus Element In2/1 -> MATLAB Function5/3(RDR)
  Bus Element In/1 -> MATLAB Function2/2(el), MATLAB Function/2(el), MATLAB Function1/3(el)
  beta/1 -> MATLAB Function5/1(Beta), MATLAB Function4/2(beta), MATLAB Function3/2(beta), MATLAB Function1/2(beta)
  MATLAB Function/1(c_x) -> Bus Creator/1
  MATLAB Function1/1(c_z) -> Bus Creator/2
  alpha/1 -> MATLAB Function4/1(alpha), MATLAB Function3/1(alpha), MATLAB Function2/1(alpha), MATLAB Function/1(alpha), MATLAB Function1/1(alpha)
  Bus Creator/1 -> Scope/1, Display/1, Coef/1
  MATLAB Function2/1(c_m) -> Bus Creator/5  "c_m"
  MATLAB Function4/1(c_n) -> Bus Creator/6  "c_n"
  MATLAB Function5/1(c_y) -> Bus Creator/3  "c_y"
  MATLAB Function3/1(c_l) -> Bus Creator/4  "c_l"

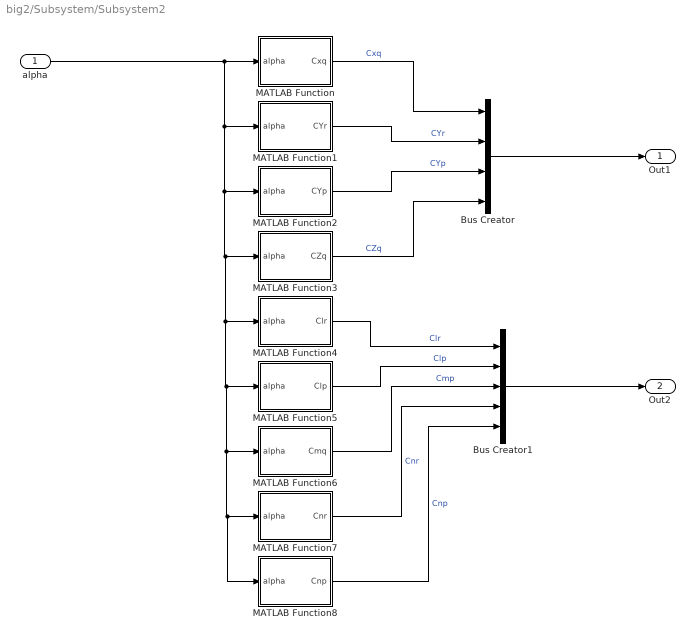
== system big2/Subsystem/Subsystem2 ==
  alpha : Inport
  Bus Creator : BusCreator  Inputs=4
  Bus Creator1 : BusCreator  Inputs=5
  MATLAB Function : MATLAB Function  TreatAsAtomicUnit=on
  MATLAB Function1 : MATLAB Function  TreatAsAtomicUnit=on
  MATLAB Function2 : MATLAB Function  TreatAsAtomicUnit=on
  MATLAB Function3 : MATLAB Function  TreatAsAtomicUnit=on
  MATLAB Function4 : MATLAB Function  TreatAsAtomicUnit=on
  MATLAB Function5 : MATLAB Function  TreatAsAtomicUnit=on
  MATLAB Function6 : MATLAB Function  TreatAsAtomicUnit=on
  MATLAB Function7 : MATLAB Function  TreatAsAtomicUnit=on
  MATLAB Function8 : MATLAB Function  TreatAsAtomicUnit=on
  Out1 : Outport
  Out2 : Outport  Port=2
  wires:
  MATLAB Function4/1(Clr) -> Bus Creator1/1  "Clr"
  MATLAB Function/1(Cxq) -> Bus Creator/1  "Cxq"
  MATLAB Function6/1(Cmq) -> Bus Creator1/3  "Cmp"
  alpha/1 -> MATLAB Function/1(alpha), MATLAB Function8/1(alpha), MATLAB Function7/1(alpha), MATLAB Function6/1(alpha), MATLAB Function5/1(alpha), MATLAB Function4/1(alpha), MATLAB Function3/1(alpha), MATLAB Function2/1(alpha), MATLAB Function1/1(alpha)
  MATLAB Function8/1(Cnp) -> Bus Creator1/5  "Cnp"
  MATLAB Function2/1(CYp) -> Bus Creator/3  "CYp"
  MATLAB Function5/1(Clp) -> Bus Creator1/2  "Clp"
  Bus Creator1/1 -> Out2/1
  MATLAB Function1/1(CYr) -> Bus Creator/2  "CYr"
  MATLAB Function3/1(CZq) -> Bus Creator/4  "CZq"
  Bus Creator/1 -> Out1/1
  MATLAB Function7/1(Cnr) -> Bus Creator1/4  "Cnr"

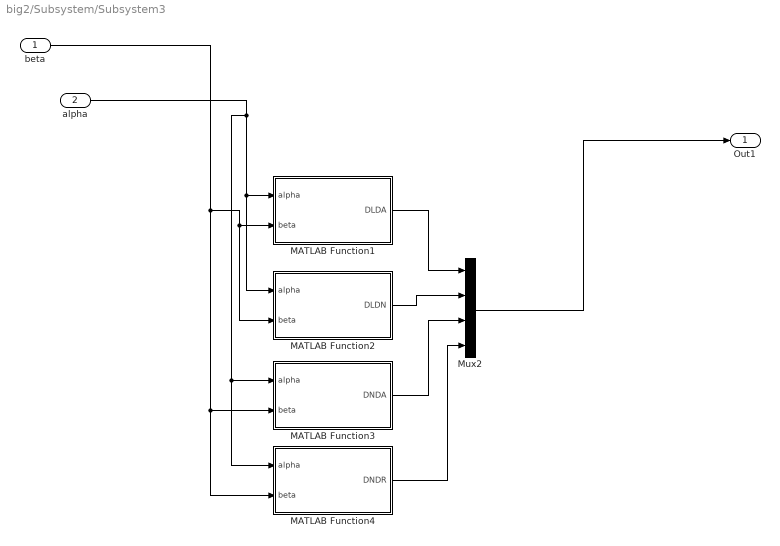
== system big2/Subsystem/Subsystem3 ==
  beta : Inport
  alpha : Inport  Port=2
  MATLAB Function1 : MATLAB Function  TreatAsAtomicUnit=on
  MATLAB Function2 : MATLAB Function  TreatAsAtomicUnit=on
  MATLAB Function3 : MATLAB Function  TreatAsAtomicUnit=on
  MATLAB Function4 : MATLAB Function  TreatAsAtomicUnit=on
  Mux2 : Mux
  Out1 : Outport
  wires:
  MATLAB Function2/1(DLDN) -> Mux2/2
  beta/1 -> MATLAB Function4/2(beta), MATLAB Function3/2(beta), MATLAB Function2/2(beta), MATLAB Function1/2(beta)
  alpha/1 -> MATLAB Function2/1(alpha), MATLAB Function1/1(alpha), MATLAB Function4/1(alpha), MATLAB Function3/1(alpha)
  Mux2/1 -> Out1/1
  MATLAB Function1/1(DLDA) -> Mux2/1
  MATLAB Function3/1(DNDA) -> Mux2/3
  MATLAB Function4/1(DNDR) -> Mux2/4

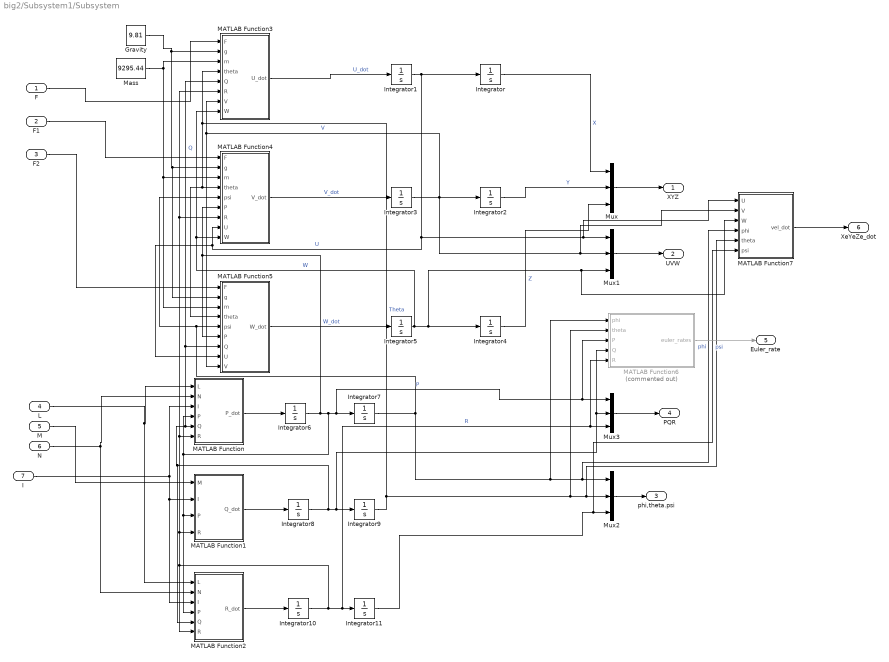
== system big2/Subsystem1/Subsystem ==
  F : Inport
  F1 : Inport  Port=2
  F2 : Inport  Port=3
  L : Inport  Port=4
  M : Inport  Port=5
  N : Inport  Port=6
  I : Inport  Port=7
  Gravity : Constant  Value=9.81
  Integrator{,2,6..8,10..11} (7 alike) : Integrator
  Integrator1 : Integrator  InitialCondition=249.99
  Integrator3 : Integrator  InitialCondition=0.01
  Integrator4 : Integrator  InitialCondition=-1500
  Integrator5 : Integrator  InitialCondition=0.5
  Integrator9 : Integrator  InitialCondition=0.002
  MATLAB Function : MATLAB Function  TreatAsAtomicUnit=on
  MATLAB Function1 : MATLAB Function  TreatAsAtomicUnit=on
  MATLAB Function2 : MATLAB Function  TreatAsAtomicUnit=on
  MATLAB Function3 : MATLAB Function  TreatAsAtomicUnit=on
  MATLAB Function4 : MATLAB Function  TreatAsAtomicUnit=on
  MATLAB Function5 : MATLAB Function  TreatAsAtomicUnit=on
  MATLAB Function6 : MATLAB Function  Commented=on  TreatAsAtomicUnit=on
  MATLAB Function7 : MATLAB Function  TreatAsAtomicUnit=on
  Mass : Constant  Value=9295.44
  Mux{,1..3} (4 alike) : Mux  Inputs=3
  XYZ : Outport
  UVW : Outport  Port=2
  phi,theta.psi : Outport  Port=3
  PQR : Outport  Port=4
  Euler_rate : Outport  Port=5
  XeYeZe_dot : Outport  Port=6
  wires:
  Gravity/1 -> MATLAB Function5/2(g), MATLAB Function4/2(g), MATLAB Function3/2(g)
  Integrator3/1 -> MATLAB Function5/9(V), MATLAB Function3/7(V), MATLAB Function7/2(V), Mux1/2, Integrator2/1  "V"
  Mass/1 -> MATLAB Function3/3(m), MATLAB Function5/3(m), MATLAB Function4/3(m)
  Integrator6/1 -> MATLAB Function/4(P), MATLAB Function2/4(P), MATLAB Function1/3(P), MATLAB Function6/3(P), Mux3/1, Integrator7/1, MATLAB Function5/6(P), MATLAB Function4/6(P)  "P"
  Integrator5/1 -> MATLAB Function7/3(W), Mux1/3, Integrator4/1, MATLAB Function4/9(W), MATLAB Function3/8(W)  "W"
  MATLAB Function/1(P_dot) -> Integrator6/1
  Integrator10/1 -> MATLAB Function2/6(R), MATLAB Function4/7(R), MATLAB Function3/6(R), MATLAB Function/6(R), MATLAB Function1/4(R), MATLAB Function6/5(R), Mux3/3, Integrator11/1  "R"
  MATLAB Function1/1(Q_dot) -> Integrator8/1
  I/1 -> MATLAB Function/3(I), MATLAB Function2/3(I), MATLAB Function1/2(I)
  Integrator1/1 -> MATLAB Function7/1(U), Mux1/1, MATLAB Function5/8(U), MATLAB Function4/8(U), Integrator/1  "U"
  Integrator9/1 -> MATLAB Function6/2(theta), MATLAB Function7/5(theta), Mux2/2, MATLAB Function5/4(theta), MATLAB Function4/4(theta), MATLAB Function3/4(theta)  "Theta"
  N/1 -> MATLAB Function/2(N), MATLAB Function2/2(N)
  Integrator8/1 -> MATLAB Function2/5(Q), MATLAB Function5/7(Q), MATLAB Function3/5(Q), MATLAB Function/5(Q), MATLAB Function6/4(Q), Mux3/2, Integrator9/1  "Q"
  Integrator11/1 -> MATLAB Function7/6(psi), Mux2/3  "psi"
  MATLAB Function2/1(R_dot) -> Integrator10/1
  F/1 -> MATLAB Function3/1(F)
  MATLAB Function3/1(U_dot) -> Integrator1/1  "U_dot"
  L/1 -> MATLAB Function2/1(L), MATLAB Function/1(L)
  F1/1 -> MATLAB Function4/1(F)
  MATLAB Function5/1(W_dot) -> Integrator5/1  "W_dot"
  MATLAB Function4/1(V_dot) -> Integrator3/1  "V_dot"
  Integrator2/1 -> Mux/2  "Y"
  Integrator4/1 -> Mux/3  "Z"
  M/1 -> MATLAB Function1/1(M)
  Integrator/1 -> Mux/1  "X"
  Integrator7/1 -> MATLAB Function5/5(psi), MATLAB Function4/5(psi), MATLAB Function6/1(phi), MATLAB Function7/4(phi), Mux2/1  "phi"
  F2/1 -> MATLAB Function5/1(F)
  Mux/1 -> XYZ/1
  Mux1/1 -> UVW/1
  Mux2/1 -> phi,theta.psi/1
  Mux3/1 -> PQR/1
  MATLAB Function6/1(euler_rates) -> Euler_rate/1
  MATLAB Function7/1(vel_dot) -> XeYeZe_dot/1

== matlab function big2/Subsystem1/Subsystem/MATLAB Function1 ==
  data: M input; Q_dot output; I input; P input; R input
function Q_dot = fcn(M,I,P,R)
    % Extract inertia components from the 3x3 inertia matrix
    Ixx = I(1,1);
    Iyy = I(2,2);
    Izz = I(3,3);
    Ixz = I(1,3); % Assuming symmetric matrix
    
    % Compute Q_dot
    Q_dot = (M + (Izz - Ixx) * P * R - Ixz * (P^2 - R^2)) / Iyy;

== matlab function big2/Subsystem1/Subsystem/MATLAB Function2 ==
  data: L input; N input; R_dot output; I input; P input; Q input; R input
function R_dot = fcn(L,N,I,P,Q,R)
    % Extract inertia components from the 3x3 inertia matrix
    Ixx = I(1,1);
    Iyy = I(2,2);
    Izz = I(3,3);
    Ixz = I(1,3); % Assuming symmetric matrix
    
    % Compute Gamma
    Gamma = Ixx * Izz - Ixz^2;

    % Compute R_dot
    R_dot = (Ixx * N + Ixz * L - (Ixx * (Ixx - Iyy) + Ixz^2) * P * Q ...
             + Ixz * (Ixx - Iyy + Izz) * Q * R) / Gamma;

    % R_dot = (Ixx * N) / Gamma;

== matlab function big2/Subsystem1/Subsystem/MATLAB Function3 ==
  data: F input; U_dot output; g input; m input; theta input; Q input; R input; V input; W input
function U_dot = fcn(F,g,m,theta,Q,R,V,W)
U_dot = R*V - Q*W - g*sin(theta) + F/m;
